simulink model "PitchAxisControlDesignModel"  (R2021b)
settings: Solver=VariableStepAuto  StartTime=0.0  StopTime=10  RelTol=1e-3
undefined symbols (not defined in the file or in its folder): den, den1, num, num1
settings Model: Creator=rfaie  LastModifiedBy=mo112

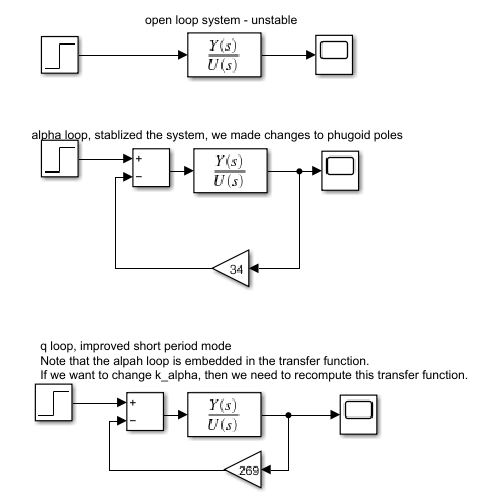
[thumbnail: Simulink's stored preview of the top-level diagram]
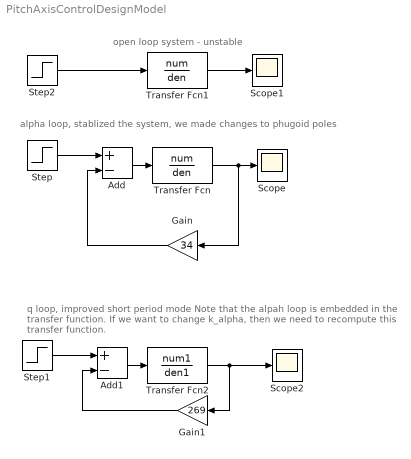
== system PitchAxisControlDesignModel ==
  note: q loop, improved short period mode
      | Note that the alpah loop is embedded in the transfer function.
      | If we want to change k_alpha, then we need to recompute this transfer function.
  note: alpha loop, stablized the system, we made changes to phugoid poles
  note: open loop system - unstable
  Add : Sum  Inputs=+-
  Add1 : Sum  Inputs=+-
  Gain : Gain  Gain=34
  Gain1 : Gain  Gain=269
  Scope : Scope
  Scope1 : Scope
  Scope2 : Scope
  Step : Step  SampleTime=0
  Step1 : Step  SampleTime=0
  Step2 : Step  SampleTime=0
  Transfer Fcn : TransferFcn  Numerator=num  Denominator=den
  Transfer Fcn1 : TransferFcn  Numerator=num  Denominator=den
  Transfer Fcn2 : TransferFcn  Numerator=num1  Denominator=den1
  wires:
  Transfer Fcn/1 -> Gain/1, Scope/1
  Add/1 -> Transfer Fcn/1
  Step/1 -> Add/1
  Gain/1 -> Add/2
  Transfer Fcn1/1 -> Scope1/1
  Add1/1 -> Transfer Fcn2/1
  Step1/1 -> Add1/1
  Transfer Fcn2/1 -> Scope2/1, Gain1/1
  Gain1/1 -> Add1/2
  Step2/1 -> Transfer Fcn1/1
